simulink model "Actividad1_P1"  (R2025b)
settings: Solver=VariableStepAuto  StartTime=0.0  StopTime=100  RelTol=1e-3
undefined symbols (not defined in the file): a, b, m
settings Model: Creator=kaoss  LastModifiedBy=kaoss

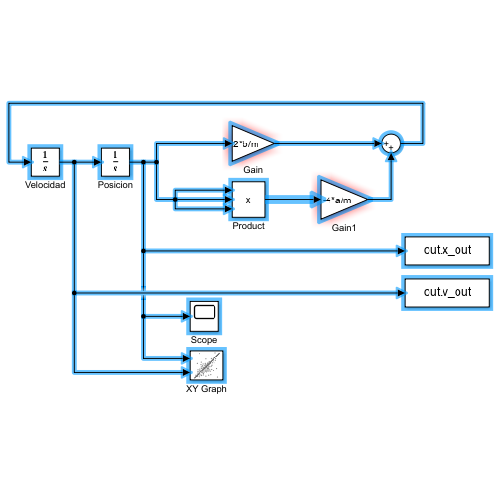
[thumbnail: Simulink's stored preview of the top-level diagram]
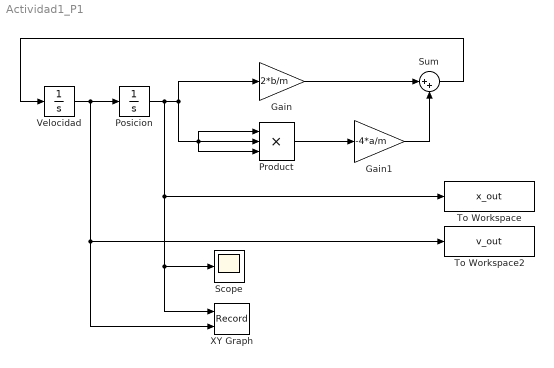
== system Actividad1_P1 ==
  Gain : Gain  Gain=2*b/m
  Gain1 : Gain  Gain=-4*a/m
  Posicion : Integrator  InitialCondition=-1.5
  Product : Product  Inputs=3
  Scope : Scope
      settings: ActiveDisplayYMinimum=-1  ActiveDisplayYMaximum=1
  Sum : Sum  Inputs=|++
  To Workspace : ToWorkspace  VariableName=x_out  SaveFormat=Structure With Time  SampleTime=-1
  To Workspace2 : ToWorkspace  VariableName=v_out  SaveFormat=Structure With Time  SampleTime=-1
  Velocidad : Integrator
  XY Graph : Record  NumPorts=2.0  FileSettingsInternal="{\"entries\":[{\"content\":{\"excelSettings\":{\"content\":{},\"type\":\"Streamout.ExcelSettings\"},\"parquetSettings\":{\"content\":{},\"type\":\"Streamout.ParquetSettings\"}},\"type\":\"Streamout.FileSettingStorage\",\"uuid\":\"\"}],\"packageUris\":[\"http:\\/\\/schema.mathworks.com\\/mf0\\/streamout_blocks\\/R2020a\"],\"version\":\"1.0\"}"  FrameSettings=[0, 0]  Layout=[1 1]  SignalsInternal="{\"entries\":[{\"content\":{\"signals\":[{\"content\":{\"blockPath\":[],\"dimensions\":[1],\"domain\":\"\",\"lineColor\":\"#a2142f\",\"plots\":[ 1 ],\"port\":1,\"sid\":[\"\"],\"signalID\":1,\"signalName\":\"Posicion\"},\"type\":\"RecordBlkView.Signal\",\"uuid\":\"\"},{\"content\":{\"blockPath\":[],\"dimensions\":[1],\"domain\":\"\",\"lineColor\":\"#139fff\",\"plots\":[ 1 ],\"port\":2,\"sid\":[\"\"],\"signalID\":2,\"signalName\":\"Velocidad\"},\"type\":\"RecordBlkView.Signal\",\"uuid\":\"\"}]},\"type\":\"RecordBlkView.InputSignals\",\"uuid\":\"\"}],\"packageUris\":[\"http:\\/\\/schema.mathworks.com\\/mf0\\/streamout_blocks\\/R2020a\"],\"version\":\"1.0\"}"  VisualizationBindings="{\"xyplotplugin\":{\"info\":[{\"series\":[{\"bindingParametersList\":[{\"parameter\":\"X-Axis\",\"signalID\":1,\"signalName\":\"Posicion\"},{\"parameter\":\"Y-Axis\",\"signalID\":2,\"signalName\":\"Velocidad\"}],\"seriesID\":0}],\"subplotID\":1}]}}"  CompatibilityTag=XY
  wires:
  Posicion/1 -> To Workspace/1, Scope/1, XY Graph/1, Product/3, Product/2, Product/1, Gain/1
  Sum/1 -> Velocidad/1
  Velocidad/1 -> To Workspace2/1, XY Graph/2, Posicion/1
  Gain/1 -> Sum/1
  Gain1/1 -> Sum/2
  Product/1 -> Gain1/1
